simulink model "euler_to_quaternion"  (R2025a)
settings: Solver=VariableStepAuto  StartTime=0.0  StopTime=1  RelTol=1e-3
values from neighbouring files (symbols this model uses):
  init_phi = init_euler(1)    [setup_data_for_DC_input_comparison_test.m]
  init_psi = init_euler(3)    [setup_data_for_DC_input_comparison_test.m]
  init_theta = init_euler(2)    [setup_data_for_DC_input_comparison_test.m]
libraries: libAxisTransformations x1
settings Model: Creator=alhallmark  LastModifiedBy=alhallmark

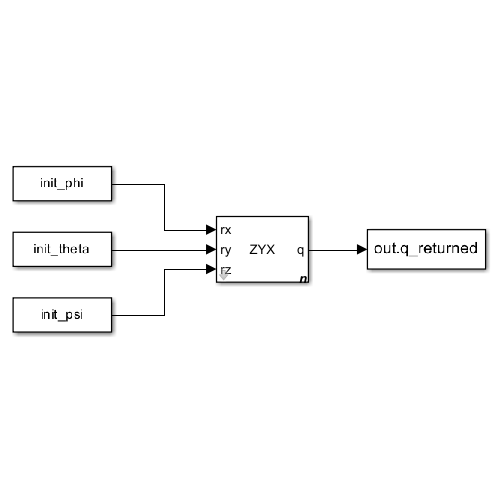
[thumbnail: Simulink's stored preview of the top-level diagram]
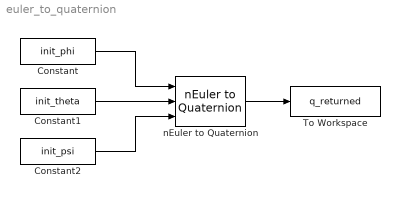
== system euler_to_quaternion ==
  Constant : Constant  Value=init_phi
  Constant1 : Constant  Value=init_theta
  Constant2 : Constant  Value=init_psi
  To Workspace : ToWorkspace  VariableName=q_returned  SampleTime=-1
      settings: MaxDataPoints=1
  nEuler to Quaternion : libAxisTransformations/nEuler to Quaternion  RotOrd=ZYX  n=1
  wires:
  Constant/1 -> nEuler to Quaternion/1
  Constant1/1 -> nEuler to Quaternion/2
  Constant2/1 -> nEuler to Quaternion/3
  nEuler to Quaternion/1 -> To Workspace/1
